simulink model "Simulink_Model"  (R2018b)
settings: Solver=VariableStepAuto  StartTime=0.0  StopTime=10.0  RelTol=1e-3
values from neighbouring files (symbols this model uses):
  Ts = 0.4    [PlanningControlRoboticArm.m]
libraries: mpclib x1
settings Model: Creator=Indiana  LastModifiedBy=jdeka

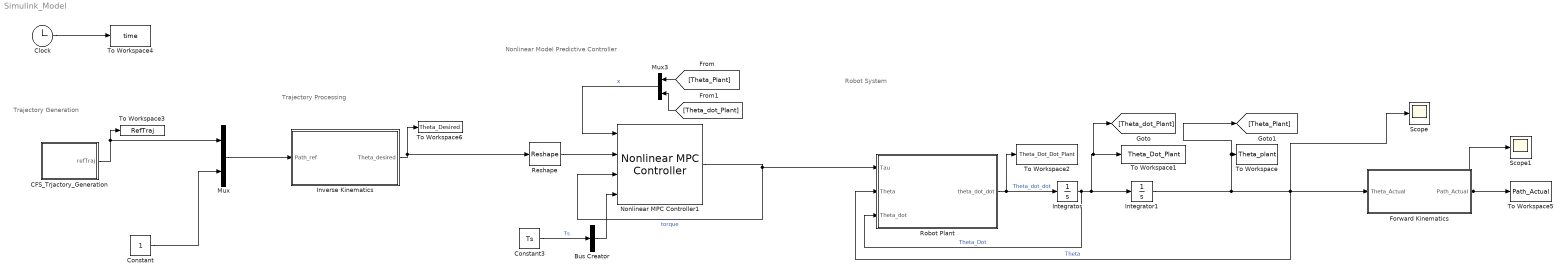
== system Simulink_Model ==
  note: Trajectory Generation
  note: Trajectory Processing
  note: Robot System
  note: Nonlinear Model Predictive Controller
  Bus Creator : BusCreator  Inputs=1  OutDataTypeStr=Bus: myBusObject_2  NonVirtualBus=on
      settings: InheritFromInputs=off
  CFS_Trjactory_Generation : MATLAB Function  TreatAsAtomicUnit=on
  Clock : Clock
  Constant : Constant
  Constant3 : Constant  Value=Ts
  Forward Kinematics : MATLAB Function  TreatAsAtomicUnit=on
  Integrator : Integrator
  Integrator1 : Integrator
  Inverse Kinematics : MATLAB Function  TreatAsAtomicUnit=on
  Mux : Mux  Inputs=2
  Mux3 : Mux  Inputs=2
  Nonlinear MPC Controller1 : mpclib/Nonlinear MPC Controller  SCDEnableBlockLinearizationSpecification=on  nlmpcobj=nlobj  UseObjectTs=on  md_enabled=off  param_enabled=on  cost_enabled=off  mvseq_enabled=off  stateseq_enabled=off  ovseq_enabled=off  slack_enabled=off  status_enabled=off  ov_min=off  ov_max=off  mv_min=off  mv_max=off  mvrate_min=off  mvrate_max=off  state_min=off  state_max=off  ov_weight=off  mv_weight=off  mvrate_weight=off  ecr_weight=off  mvtarget_enabled=off  nlp_initialize=off
      settings: SourceProductName=Model Predictive Control Toolbox
  Reshape : Reshape  OutputDimensionality=Row vector (2-D)
  Robot Plant : MATLAB Function  TreatAsAtomicUnit=on
  Scope : Scope
  Scope1 : Scope
  To Workspace : ToWorkspace  VariableName=Theta_plant  SampleTime=-1
  To Workspace1 : ToWorkspace  VariableName=Theta_Dot_Plant  SampleTime=-1
  To Workspace2 : ToWorkspace  VariableName=Theta_Dot_Dot_Plant  SampleTime=-1
  To Workspace3 : ToWorkspace  VariableName=RefTraj  SampleTime=-1
  To Workspace4 : ToWorkspace  VariableName=time  SampleTime=-1
  To Workspace5 : ToWorkspace  VariableName=Path_Actual  SampleTime=-1
  To Workspace6 : ToWorkspace  VariableName=Theta_Desired  SampleTime=-1
  wires:
  Robot Plant/1(theta_dot_dot) -> To Workspace2/1, Integrator/1  "Theta_dot_dot"
  Integrator/1 -> [Theta_dot_Plant], To Workspace1/1, Integrator1/1, Robot Plant/3(Theta_dot)  "Theta_Dot"
  Integrator1/1 -> [Theta_Plant], To Workspace/1, Forward Kinematics/1(Theta_Actual), Robot Plant/2(Theta), Scope/1  "Theta"
  Clock/1 -> To Workspace4/1
  Forward Kinematics/1(Path_Actual) -> Scope1/1, To Workspace5/1
  CFS_Trjactory_Generation/1(refTraj) -> To Workspace3/1, Mux/1
  Bus Creator/1 -> Nonlinear MPC Controller1/4
  Mux3/1 -> Nonlinear MPC Controller1/1  "x"
  Inverse Kinematics/1(Theta_desired) -> To Workspace6/1, Reshape/1
  Reshape/1 -> Nonlinear MPC Controller1/2
  Constant3/1 -> Bus Creator/1  "Ts"
  Nonlinear MPC Controller1/1 -> Robot Plant/1(Tau), Nonlinear MPC Controller1/3  "torque"
  [Theta_Plant] -> Mux3/1
  [Theta_dot_Plant] -> Mux3/2
  Constant/1 -> Mux/2
  Mux/1 -> Inverse Kinematics/1(Path_ref)

== matlab function Simulink_Model/CFS_Trjactory_Generation ==
  data: refTraj output
function refTraj = fcn()

% This script specifies the planning problem

nstep = 60; % number of sampling points on the path
dim = 2; % dimention of the problem, default 2
dt = 1; % sampling time (s)
start = [0;0]; % starting point
ending = [9;0]; % ending point
margin = 0.25; % safety margin

%% Initialize the path by linear interpolation
path = [];
for i = 1:nstep
    path(:,i) = (nstep-i)/(nstep-1)*start+(i-1)/(nstep-1)*ending;
end
refpath = [];
for i=1:nstep
    refpath = [refpath;path(:,i)];
end
oripath = refpath;
%% Initialize the obstacles
nobj = 5;
obs = {};

obs{1}.v = [0;0]; % velocity of the obstacle
obs{1}.poly = [2 4.3 4 3;3 3 -1 -1]; % shape of the obstacle
obs{2}.v = [0;0];
obs{2}.poly = [6 7 7.5 6;0 1 -3 -3];
obs{3}.v = [0;0];
obs{3}.poly = [1 2 1.5 0;-2 -3 -0.1 -1];
obs{4}.v = [0;0];
obs{4}.poly = [1 6 1 5; 1 1 2 2];
obs{5}.v = [0;0];
obs{5}.poly = [3 7 7 3;-3 -3 -2.1 -2.1];


%% The cost function
% The distance metric between the original path and the new path
Q1 = eye(nstep*dim);
% The velocity
Vdiff = eye(nstep*dim)-diag(ones(1,(nstep-1)*dim),dim);
Q2 = Vdiff(1:(nstep-1)*dim,:)'*Q1(1+dim:end,1+dim:end)*Vdiff(1:(nstep-1)*dim,:);
% The accelaration
Adiff = Vdiff-diag(ones(1,(nstep-1)*dim),dim)+diag(ones(1,(nstep-2)*dim),dim*2);
Q3 = Adiff(1:(nstep-2)*dim,:)'*Adiff(1:(nstep-2)*dim,:);
% The weight
cref = [0,0,0];
cabs = [0,0,1];
% The total costj
Qref = Q1*cref(1)/nstep+Q2*cref(2)*(nstep-1)+Q3*cref(3)*(nstep-1)^4/(nstep-2);
Qabs = Q1*cabs(1)/nstep+Q2*cabs(2)*(nstep-1)+Q3*cabs(3)*(nstep-1)^4/(nstep-2);

%% The boundary constraint
Aeq = zeros(4*dim,nstep*dim+nstep);
Aeq(0*dim+1:1*dim,1:dim) = eye(dim);
Aeq(1*dim+1:2*dim,(nstep-1)*dim+1:nstep*dim) = eye(dim);
Aeq(2*dim+1:3*dim,1:2*dim) = [-eye(dim) eye(dim)];
Aeq(3*dim+1:4*dim,(nstep-2)*dim+1:nstep*dim) = [-eye(dim) eye(dim)];
beq = [path(:,1);path(:,end);path(:,2)-path(:,1);path(:,end)-path(:,end-1)];


%%
% This script implements the CFS algorithm to solve a problem specified in
% problem.m

clear all, clc 


addpath('lib')

%% Initialize the problem
problem

%% The Iteration
MAX_ITER = 100;

figure; hold on

tic
for k = 1:MAX_ITER
    % The constraints
    Lstack = []; Sstack = [];
    for i=1:nstep
        for j=1:nobj
            poly = obs{j}.poly+obs{j}.v*ones(1,4)*dt*i;
            [L,S,d] = d2poly(refpath((i-1)*dim+1:i*dim)',poly');
            Lstack = [Lstack;zeros(1,(i-1)*dim) L zeros(1,(nstep-i)*dim) zeros(1,nstep)];
            Sstack = [Sstack;S-margin];
        end
    end
    % QP
    Qe = Qref+Qabs;
    soln = quadprog(Qe,-Qref*oripath,Lstack(:,1:size(Qe,1)),Sstack,Aeq(:,1:size(Qe,1)),beq);
    
    pathnew = soln(1:dim*nstep);
    diff = norm(refpath-pathnew);
    if diff < 0.001*nstep*(dim)
        disp(['converged at step ',num2str(k)]);
        break
    end
    refpath = pathnew;
    plot(pathnew(1:dim:end),pathnew(2:dim:end))
end
%% Statistics
time = toc
disp(['final cost: ']);
cost_quadratic(pathnew,oripath,Qref,Qabs)




refTraj ;

== matlab function Simulink_Model/Robot Plant ==
  data: Tau input; theta_dot_dot output; Theta input; Theta_dot input
function theta_dot_dot = fcn(Tau, Theta, Theta_dot)
%% Variables 

theta1 = Theta(1); 
theta2 = Theta(2); 
theta3 = Theta(3); 

theta1_dot = Theta_dot(1) ;
theta2_dot = Theta_dot(2);
theta3_dot = Theta_dot(3);

%%  EOM Parameters : 
m1 = 182.5591;
m2 = 121.4263;
m3 = 28.4126+16.4793;
L1 = 1.045;
L2 = 1.3;
L3 = 1.025+.29;

%R1 =1; 

g = 9.81; % Acceleration Due to Gravity 
%%
%Mass Matrix Parameter Construction
%Changed 'R1' to 'L1'
M_11 = .5*m1*(L1)^2 + (1/3)*m2*(L2)^2*(cos(theta2))^2 +(1/3)*m3*(L3)^2*cos(theta2+theta3) + m3*(L2)^2*(cos(theta2))^2 + m3*L2*L3*cos(theta2+theta3)*cos(theta2);
M_12 =0 ; 
M_13 =0 ;
M_21 =0 ;
M_22 = (1/3)*m2*(L2)^2 + (1/3)*m3*(L3)^2 + m3*(L2)^2 + m3*L2*L3*cos(theta3);
M_23 = (1/3)*m3*(L3)^2 + m3*(L2)^2 + (1/3)*m3*L2*L3*cos(theta3);
M_31 = 0; 
M_32 = (1/3)*m3*(L3)^2 + m3*(L2)^2 + (1/3)*m3*L2*L3*cos(theta3);
M_33 = (1/3)*m3*(L3)^2; 

% Coriolis Matrix Parameter Construction: 

C_11 = (-(4/3)*m2*(L2)^2*sin(2*theta2)-(1/3)*m3*(L3)^2*sin(2*(theta2+theta3))-m3*L2*L3*sin(2*theta2 + theta3))*theta2_dot*theta1_dot +(-(1/3)*m3*(L2)^2*sin(2*(theta2+theta3)-m3*L2*L3*cos(theta2)*sin(theta2+theta3)))*theta3_dot*theta1_dot ; 
C_21 = (-m3*L2*L3*sin(theta3))*theta2_dot*theta3_dot + (-(1/2)*m3*L2*L3*sin(theta3))*(theta3_dot)^2 + ((1/6)*m2*(L2)^2*sin(2*theta2) + (1/6)*m3*(L3)^2*sin(2*(theta2+theta3)) + (1/2)*m3*(L2)^2*sin(2*theta2) + (1/2)*m3*L2*L3*sin(2*theta2+theta3))*(theta1_dot)^2; 
C_31 = ((1/2)*m3*L2*L3*sin(theta3))*(theta2_dot)^2 + ((1/6)*m3*(L3)^2*sin(2*(theta2+theta3)) + (1/2)*m3*L2*L3*cos(theta2)*sin(theta2+theta3))*(theta1_dot)^2; 


% Gravity Matrix Parameter Construction: 
G_11 = 0; 
G_21 = .5*m2*g*L2*cos(theta2) + .5*m3*g*L3*cos(theta2+theta3) + m3*g*L2*cos(theta2); 
G_31 = .5*m3*g*L3*cos(theta2+theta3); 

%% Differential EOM: 

%Mass Matrix: 
M = [M_11, M_12, M_13; 
     M_21, M_22, M_23; 
     M_31, M_32, M_33];
% Coriolis Matrix: 
C = [C_11;C_21;C_31];
%Gravity Matrix: 
G = [G_11;G_21;G_31]; 

theta_dot_dot = inv(M)*(Tau-C-G);

== matlab function Simulink_Model/Inverse Kinematics ==
  data: Path_ref input; Theta_desired output
function Theta_desired = fcn(Path_ref)

%Imported from CFS Code
P_x = Path_ref(:,1); 
P_y = Path_ref(:,2);
% Probably Kept Constant (CFS code is 2D and Does not include Z coordinate)
P_z = Path_ref(:,3); 

theta1 = atan2(P_y,P_x); 
r = +- sqrt((P_x)^2+(P_y)^2); 
D = +-sqrt((P_z-L1)^2+(r)^2); 
theta3 = acos((D^2-L3^2-L2^2)/(2*L2*L3)); 
% theta3 = acos(((P_z-L1)^2+P_x^2+P_y^2-L3^2-L2^2)/(2*L2*L3));
theta2 = atan2(r,P_z-1)-atan2(L2+L3*cos(theta3),L3*sin(theta3));


Theta_desired = [theta1,theta2,theta3];

== matlab function Simulink_Model/Forward Kinematics ==
  data: Theta_Actual input; Path_Actual output
function Path_Actual = fcn(Theta_Actual)

theta1 = Theta_Actual(1); 
theta2 = Theta_Actual(2); 
theta3 = Theta_Actual(3); 

P_x = (L2*cos(theta2) + L3*cos(theta2+theta3))*sin(theta1); 
P_y = (L2*cos(theta2) + L3*cos(theta2+theta3))*cos(theta1); 
P_z = L2*sin(theta2) + L3*sin(theta2+theta3) + L1; 


Path_Actual = [P_x, P_y,P_z];
